simulink model "optimal_servo_without_ff"  (R2019b)
settings: Solver=VariableStepAuto  StartTime=0.0  StopTime=10.0  RelTol=1e-3
values from neighbouring files (symbols this model uses):
  A = [0 1 0 0 ... (first row only)    [following.m]    (also in following2.m; observer.m; opt_servo.m; optimal_care.m = [0 1)
  B = [0 ... (first row only)    [following.m]    (also in following2.m; observer.m; opt_servo.m; optimal_care.m)
  C = [0 0 1 0]    [following.m]    (also in following2.m; observer.m; opt_servo.m)
  Fa = [-K+2*G*inv(P22)*P12' 1]*inv(M0)*[zeros(4,1); 1]    [opt_servo.m]
  Fb = -2*G*inv(P22)*P12'    [opt_servo.m]
  G = Ke(5)    [following2.m]    (also in opt_servo.m = -inv(Re)*B'*P12; pidtest.m = 1/(s^2+s+1))
  K = -acker(A,B,p)    [following.m]    (also in following2.m = Ke(1:4); observer.m; opt_servo.m = -inv(Re)*B'*P11; optimal_care.m = -inv(R)*B'*P)
  x0 = zeros(4,1)    [following.m]    (also in following2.m; observer.m = [-0.5 0 0.5 0]'; opt_servo.m = [ 0 0 0.25 0 ]'; optimal_care.m = [1)
settings Model: Creator=shohei  LastModifiedBy=shohei

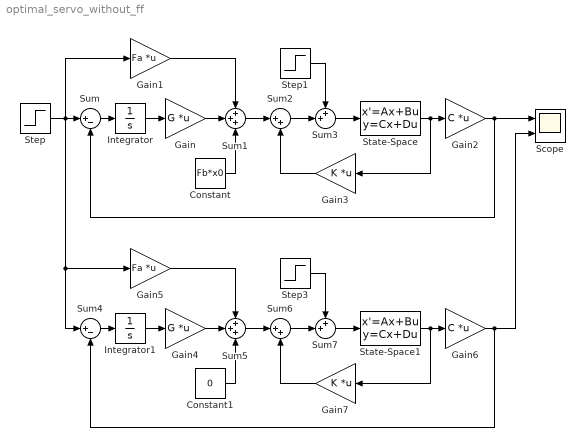
== system optimal_servo_without_ff ==
  Constant : Constant  Value=Fb*x0
  Constant1 : Constant  Value=0
  Gain : Gain  Gain=G  Multiplication=Matrix(K*u)
  Gain1 : Gain  Gain=Fa  Multiplication=Matrix(K*u)
  Gain2 : Gain  Gain=C  Multiplication=Matrix(K*u)
  Gain3 : Gain  Gain=K  Multiplication=Matrix(K*u)
  Gain4 : Gain  Gain=G  Multiplication=Matrix(K*u)
  Gain5 : Gain  Gain=Fa  Multiplication=Matrix(K*u)
  Gain6 : Gain  Gain=C  Multiplication=Matrix(K*u)
  Gain7 : Gain  Gain=K  Multiplication=Matrix(K*u)
  Integrator : Integrator
  Integrator1 : Integrator
  Scope : Scope  NumInputPorts=2
  State-Space : StateSpace  A=A  B=B  C=eye(4)  D=zeros(4,1)  InitialCondition=x0
  State-Space1 : StateSpace  A=A  B=B  C=eye(4)  D=zeros(4,1)  InitialCondition=x0
  Step : Step  SampleTime=0
  Step1 : Step  Time=5  SampleTime=0
  Step3 : Step  Time=5  SampleTime=0
  Sum : Sum  Inputs=|+-
  Sum1 : Sum  Inputs=+++
  Sum2 : Sum  Inputs=|++
  Sum3 : Sum  Inputs=++|
  Sum4 : Sum  Inputs=|+-
  Sum5 : Sum  Inputs=+++
  Sum6 : Sum  Inputs=|++
  Sum7 : Sum  Inputs=++|
  wires:
  Gain/1 -> Sum1/2
  Step/1 -> Sum4/1, Gain5/1, Gain1/1, Sum/1
  Sum/1 -> Integrator/1
  Sum6/1 -> Sum7/2
  Integrator/1 -> Gain/1
  Sum1/1 -> Sum2/1
  Gain4/1 -> Sum5/2
  Constant/1 -> Sum1/3
  State-Space1/1 -> Gain7/1, Gain6/1
  Sum3/1 -> State-Space/1
  Integrator1/1 -> Gain4/1
  Sum7/1 -> State-Space1/1
  Constant1/1 -> Sum5/3
  Sum5/1 -> Sum6/1
  Step1/1 -> Sum3/1
  State-Space/1 -> Gain3/1, Gain2/1
  Sum2/1 -> Sum3/2
  Gain1/1 -> Sum1/1
  Gain5/1 -> Sum5/1
  Gain2/1 -> Sum/2, Scope/1
  Gain3/1 -> Sum2/2
  Gain7/1 -> Sum6/2
  Gain6/1 -> Scope/2, Sum4/2
  Sum4/1 -> Integrator1/1
  Step3/1 -> Sum7/1
